simulink model "SRSCrt_MdSwXX_Stat_67_2"  (R2018b)
settings: Solver=FixedStepDiscrete  StartTime=0.0  StopTime=10.0  FixedStep=0.01  RelTol=1e-3
undefined symbols (not defined in the file or in its folder): KeSMSbSRSPosNumConfig_Val
settings Model: Creator=sn2xws  LastModifiedBy=sn2xws
settings DataIOCC: SaveFormat=StructureWithTime
settings OptimizationCC: DefaultParameterBehavior=Inlined  EnhancedBackFolding=on  PassReuseOutputArgsAs=Individual arguments  ZeroExternalMemoryAtStartup=off  ZeroInternalMemoryAtStartup=off  OptimizeBlockOrder=speed  DifferentSizesBufferReuse=on  OptimizationCustomize=off
settings DebuggingCC: ParameterTunabilityLossMsg=error
settings ModelReferenceCC: ModelReferenceNumInstancesAllowed=Single
settings SFSimCC: MATLABDynamicMemAlloc=off
settings RTWCC: SystemTargetFile=autosar.tlc  GenCodeOnly=on  TemplateMakefile=ert_default_tmf  Description=AUTOSAR  GenerateReport=on  IncludeHyperlinkInReport=on  LaunchReport=on  GenerateTraceInfo=on  GenerateTraceReport=on  GenerateTraceReportSl=on  GenerateTraceReportSf=on  GenerateTraceReportEml=on
settings CodeAppCC: ForceParamTrailComments=on  IgnoreCustomStorageClasses=off  OperatorAnnotations=on  SimulinkDataObjDesc=on  SFDataObjDesc=on  InsertBlockDesc=on
settings STFCustomTargetCC: TargetLangStandard=C99 (ISO)  MultiwordLength=256  ParMdlRefBuildCompliant=on  CompOptLevelCompliant=on  IncludeMdlTerminateFcn=off  CombineOutputUpdateFcns=on  SuppressErrorStatus=on  ERTCustomFileBanners=on  SupportNonFinite=off  SupportComplex=off  SupportContinuousTime=off  SupportNonInlinedSFcns=off  RemoveResetFunc=on  MATLABClassNameForMDSCustomization=Simulink.SoftwareTarget.ERTCustomization  AutosarCompliant=on  UseToolchainInfoCompliant=on  LookupTableObjectStructAxisOrder=2,1,3,4,...  LUTObjectStructOrderEvenSpacing=Size,Table,Breakpoints  SystemTargetFile=autosar.tlc
settings ERTTargetCC: TargetLangStandard=C99 (ISO)  ConcurrentExecutionCompliant=off  IncludeMdlTerminateFcn=off  SuppressErrorStatus=on  SupportNonFinite=off  SupportComplex=off  ModelStepFunctionPrototypeControlCompliant=off  CPPClassGenCompliant=off  AutosarCompliant=on  LookupTableObjectStructAxisOrder=2,1,3,4,...  LUTObjectStructOrderEvenSpacing=Size,Table,Breakpoints  InlinedParameterPlacement=NonHierarchical  ERTCustomFileTemplate=example_file_process.tlc

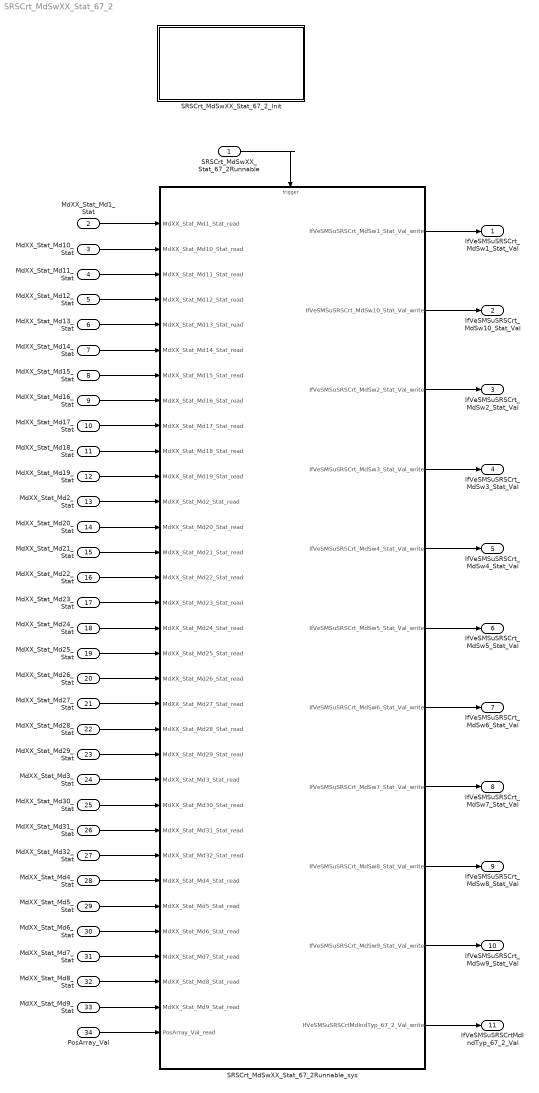
== system SRSCrt_MdSwXX_Stat_67_2 ==
  SRSCrt_MdSwXX_Stat_67_2Runnable : Inport  SampleTime=0.01  OutputFunctionCall=on
  MdXX_Stat_Md1_Stat : Inport  Port=2  OutDataTypeStr=uint8  PortDimensions=1
  MdXX_Stat_Md10_Stat : Inport  Port=3  OutDataTypeStr=uint8  PortDimensions=1
  MdXX_Stat_Md11_Stat : Inport  Port=4  OutDataTypeStr=uint8  PortDimensions=1
  MdXX_Stat_Md12_Stat : Inport  Port=5  OutDataTypeStr=uint8  PortDimensions=1
  MdXX_Stat_Md13_Stat : Inport  Port=6  OutDataTypeStr=uint8  PortDimensions=1
  MdXX_Stat_Md14_Stat : Inport  Port=7  OutDataTypeStr=uint8  PortDimensions=1
  MdXX_Stat_Md15_Stat : Inport  Port=8  OutDataTypeStr=uint8  PortDimensions=1
  MdXX_Stat_Md16_Stat : Inport  Port=9  OutDataTypeStr=uint8  PortDimensions=1
  MdXX_Stat_Md17_Stat : Inport  Port=10  OutDataTypeStr=uint8  PortDimensions=1
  MdXX_Stat_Md18_Stat : Inport  Port=11  OutDataTypeStr=uint8  PortDimensions=1
  MdXX_Stat_Md19_Stat : Inport  Port=12  OutDataTypeStr=uint8  PortDimensions=1
  MdXX_Stat_Md2_Stat : Inport  Port=13  OutDataTypeStr=uint8  PortDimensions=1
  MdXX_Stat_Md20_Stat : Inport  Port=14  OutDataTypeStr=uint8  PortDimensions=1
  MdXX_Stat_Md21_Stat : Inport  Port=15  OutDataTypeStr=uint8  PortDimensions=1
  MdXX_Stat_Md22_Stat : Inport  Port=16  OutDataTypeStr=uint8  PortDimensions=1
  MdXX_Stat_Md23_Stat : Inport  Port=17  OutDataTypeStr=uint8  PortDimensions=1
  MdXX_Stat_Md24_Stat : Inport  Port=18  OutDataTypeStr=uint8  PortDimensions=1
  MdXX_Stat_Md25_Stat : Inport  Port=19  OutDataTypeStr=uint8  PortDimensions=1
  MdXX_Stat_Md26_Stat : Inport  Port=20  OutDataTypeStr=uint8  PortDimensions=1
  MdXX_Stat_Md27_Stat : Inport  Port=21  OutDataTypeStr=uint8  PortDimensions=1
  MdXX_Stat_Md28_Stat : Inport  Port=22  OutDataTypeStr=uint8  PortDimensions=1
  MdXX_Stat_Md29_Stat : Inport  Port=23  OutDataTypeStr=uint8  PortDimensions=1
  MdXX_Stat_Md3_Stat : Inport  Port=24  OutDataTypeStr=uint8  PortDimensions=1
  MdXX_Stat_Md30_Stat : Inport  Port=25  OutDataTypeStr=uint8  PortDimensions=1
  MdXX_Stat_Md31_Stat : Inport  Port=26  OutDataTypeStr=uint8  PortDimensions=1
  MdXX_Stat_Md32_Stat : Inport  Port=27  OutDataTypeStr=uint8  PortDimensions=1
  MdXX_Stat_Md4_Stat : Inport  Port=28  OutDataTypeStr=uint8  PortDimensions=1
  MdXX_Stat_Md5_Stat : Inport  Port=29  OutDataTypeStr=uint8  PortDimensions=1
  MdXX_Stat_Md6_Stat : Inport  Port=30  OutDataTypeStr=uint8  PortDimensions=1
  MdXX_Stat_Md7_Stat : Inport  Port=31  OutDataTypeStr=uint8  PortDimensions=1
  MdXX_Stat_Md8_Stat : Inport  Port=32  OutDataTypeStr=uint8  PortDimensions=1
  MdXX_Stat_Md9_Stat : Inport  Port=33  OutDataTypeStr=uint8  PortDimensions=1
  PosArray_Val : Inport  Port=34  OutDataTypeStr=uint8  PortDimensions=11
  SRSCrt_MdSwXX_Stat_67_2Runnable_sys : Subsystem
  SRSCrt_MdSwXX_Stat_67_2_Init : Subsystem
  IfVeSMSuSRSCrt_MdSw1_Stat_Val : Outport  OutDataTypeStr=uint8  PortDimensions=1
  IfVeSMSuSRSCrt_MdSw10_Stat_Val : Outport  Port=2  OutDataTypeStr=uint8  PortDimensions=1
  IfVeSMSuSRSCrt_MdSw2_Stat_Val : Outport  Port=3  OutDataTypeStr=uint8  PortDimensions=1
  IfVeSMSuSRSCrt_MdSw3_Stat_Val : Outport  Port=4  OutDataTypeStr=uint8  PortDimensions=1
  IfVeSMSuSRSCrt_MdSw4_Stat_Val : Outport  Port=5  OutDataTypeStr=uint8  PortDimensions=1
  IfVeSMSuSRSCrt_MdSw5_Stat_Val : Outport  Port=6  OutDataTypeStr=uint8  PortDimensions=1
  IfVeSMSuSRSCrt_MdSw6_Stat_Val : Outport  Port=7  OutDataTypeStr=uint8  PortDimensions=1
  IfVeSMSuSRSCrt_MdSw7_Stat_Val : Outport  Port=8  OutDataTypeStr=uint8  PortDimensions=1
  IfVeSMSuSRSCrt_MdSw8_Stat_Val : Outport  Port=9  OutDataTypeStr=uint8  PortDimensions=1
  IfVeSMSuSRSCrt_MdSw9_Stat_Val : Outport  Port=10  OutDataTypeStr=uint8  PortDimensions=1
  IfVeSMSuSRSCrtMdIndTyp_67_2_Val : Outport  Port=11  OutDataTypeStr=uint8  PortDimensions=1
  wires:
  MdXX_Stat_Md1_Stat/1 -> SRSCrt_MdSwXX_Stat_67_2Runnable_sys/1(MdXX_Stat_Md1_Stat_read)
  MdXX_Stat_Md10_Stat/1 -> SRSCrt_MdSwXX_Stat_67_2Runnable_sys/2(MdXX_Stat_Md10_Stat_read)
  MdXX_Stat_Md11_Stat/1 -> SRSCrt_MdSwXX_Stat_67_2Runnable_sys/3(MdXX_Stat_Md11_Stat_read)
  MdXX_Stat_Md12_Stat/1 -> SRSCrt_MdSwXX_Stat_67_2Runnable_sys/4(MdXX_Stat_Md12_Stat_read)
  MdXX_Stat_Md13_Stat/1 -> SRSCrt_MdSwXX_Stat_67_2Runnable_sys/5(MdXX_Stat_Md13_Stat_read)
  MdXX_Stat_Md14_Stat/1 -> SRSCrt_MdSwXX_Stat_67_2Runnable_sys/6(MdXX_Stat_Md14_Stat_read)
  MdXX_Stat_Md15_Stat/1 -> SRSCrt_MdSwXX_Stat_67_2Runnable_sys/7(MdXX_Stat_Md15_Stat_read)
  MdXX_Stat_Md16_Stat/1 -> SRSCrt_MdSwXX_Stat_67_2Runnable_sys/8(MdXX_Stat_Md16_Stat_read)
  MdXX_Stat_Md17_Stat/1 -> SRSCrt_MdSwXX_Stat_67_2Runnable_sys/9(MdXX_Stat_Md17_Stat_read)
  MdXX_Stat_Md18_Stat/1 -> SRSCrt_MdSwXX_Stat_67_2Runnable_sys/10(MdXX_Stat_Md18_Stat_read)
  MdXX_Stat_Md19_Stat/1 -> SRSCrt_MdSwXX_Stat_67_2Runnable_sys/11(MdXX_Stat_Md19_Stat_read)
  MdXX_Stat_Md2_Stat/1 -> SRSCrt_MdSwXX_Stat_67_2Runnable_sys/12(MdXX_Stat_Md2_Stat_read)
  MdXX_Stat_Md20_Stat/1 -> SRSCrt_MdSwXX_Stat_67_2Runnable_sys/13(MdXX_Stat_Md20_Stat_read)
  MdXX_Stat_Md21_Stat/1 -> SRSCrt_MdSwXX_Stat_67_2Runnable_sys/14(MdXX_Stat_Md21_Stat_read)
  MdXX_Stat_Md22_Stat/1 -> SRSCrt_MdSwXX_Stat_67_2Runnable_sys/15(MdXX_Stat_Md22_Stat_read)
  MdXX_Stat_Md23_Stat/1 -> SRSCrt_MdSwXX_Stat_67_2Runnable_sys/16(MdXX_Stat_Md23_Stat_read)
  MdXX_Stat_Md24_Stat/1 -> SRSCrt_MdSwXX_Stat_67_2Runnable_sys/17(MdXX_Stat_Md24_Stat_read)
  MdXX_Stat_Md25_Stat/1 -> SRSCrt_MdSwXX_Stat_67_2Runnable_sys/18(MdXX_Stat_Md25_Stat_read)
  MdXX_Stat_Md26_Stat/1 -> SRSCrt_MdSwXX_Stat_67_2Runnable_sys/19(MdXX_Stat_Md26_Stat_read)
  MdXX_Stat_Md27_Stat/1 -> SRSCrt_MdSwXX_Stat_67_2Runnable_sys/20(MdXX_Stat_Md27_Stat_read)
  MdXX_Stat_Md28_Stat/1 -> SRSCrt_MdSwXX_Stat_67_2Runnable_sys/21(MdXX_Stat_Md28_Stat_read)
  MdXX_Stat_Md29_Stat/1 -> SRSCrt_MdSwXX_Stat_67_2Runnable_sys/22(MdXX_Stat_Md29_Stat_read)
  MdXX_Stat_Md3_Stat/1 -> SRSCrt_MdSwXX_Stat_67_2Runnable_sys/23(MdXX_Stat_Md3_Stat_read)
  MdXX_Stat_Md30_Stat/1 -> SRSCrt_MdSwXX_Stat_67_2Runnable_sys/24(MdXX_Stat_Md30_Stat_read)
  MdXX_Stat_Md31_Stat/1 -> SRSCrt_MdSwXX_Stat_67_2Runnable_sys/25(MdXX_Stat_Md31_Stat_read)
  MdXX_Stat_Md32_Stat/1 -> SRSCrt_MdSwXX_Stat_67_2Runnable_sys/26(MdXX_Stat_Md32_Stat_read)
  MdXX_Stat_Md4_Stat/1 -> SRSCrt_MdSwXX_Stat_67_2Runnable_sys/27(MdXX_Stat_Md4_Stat_read)
  MdXX_Stat_Md5_Stat/1 -> SRSCrt_MdSwXX_Stat_67_2Runnable_sys/28(MdXX_Stat_Md5_Stat_read)
  MdXX_Stat_Md6_Stat/1 -> SRSCrt_MdSwXX_Stat_67_2Runnable_sys/29(MdXX_Stat_Md6_Stat_read)
  MdXX_Stat_Md7_Stat/1 -> SRSCrt_MdSwXX_Stat_67_2Runnable_sys/30(MdXX_Stat_Md7_Stat_read)
  MdXX_Stat_Md8_Stat/1 -> SRSCrt_MdSwXX_Stat_67_2Runnable_sys/31(MdXX_Stat_Md8_Stat_read)
  MdXX_Stat_Md9_Stat/1 -> SRSCrt_MdSwXX_Stat_67_2Runnable_sys/32(MdXX_Stat_Md9_Stat_read)
  PosArray_Val/1 -> SRSCrt_MdSwXX_Stat_67_2Runnable_sys/33(PosArray_Val_read)
  SRSCrt_MdSwXX_Stat_67_2Runnable_sys/1(IfVeSMSuSRSCrt_MdSw1_Stat_Val_write) -> IfVeSMSuSRSCrt_MdSw1_Stat_Val/1
  SRSCrt_MdSwXX_Stat_67_2Runnable_sys/2(IfVeSMSuSRSCrt_MdSw10_Stat_Val_write) -> IfVeSMSuSRSCrt_MdSw10_Stat_Val/1
  SRSCrt_MdSwXX_Stat_67_2Runnable_sys/3(IfVeSMSuSRSCrt_MdSw2_Stat_Val_write) -> IfVeSMSuSRSCrt_MdSw2_Stat_Val/1
  SRSCrt_MdSwXX_Stat_67_2Runnable_sys/4(IfVeSMSuSRSCrt_MdSw3_Stat_Val_write) -> IfVeSMSuSRSCrt_MdSw3_Stat_Val/1
  SRSCrt_MdSwXX_Stat_67_2Runnable_sys/5(IfVeSMSuSRSCrt_MdSw4_Stat_Val_write) -> IfVeSMSuSRSCrt_MdSw4_Stat_Val/1
  SRSCrt_MdSwXX_Stat_67_2Runnable_sys/6(IfVeSMSuSRSCrt_MdSw5_Stat_Val_write) -> IfVeSMSuSRSCrt_MdSw5_Stat_Val/1
  SRSCrt_MdSwXX_Stat_67_2Runnable_sys/7(IfVeSMSuSRSCrt_MdSw6_Stat_Val_write) -> IfVeSMSuSRSCrt_MdSw6_Stat_Val/1
  SRSCrt_MdSwXX_Stat_67_2Runnable_sys/8(IfVeSMSuSRSCrt_MdSw7_Stat_Val_write) -> IfVeSMSuSRSCrt_MdSw7_Stat_Val/1
  SRSCrt_MdSwXX_Stat_67_2Runnable_sys/9(IfVeSMSuSRSCrt_MdSw8_Stat_Val_write) -> IfVeSMSuSRSCrt_MdSw8_Stat_Val/1
  SRSCrt_MdSwXX_Stat_67_2Runnable_sys/10(IfVeSMSuSRSCrt_MdSw9_Stat_Val_write) -> IfVeSMSuSRSCrt_MdSw9_Stat_Val/1
  SRSCrt_MdSwXX_Stat_67_2Runnable_sys/11(IfVeSMSuSRSCrtMdIndTyp_67_2_Val_write) -> IfVeSMSuSRSCrtMdIndTyp_67_2_Val/1
  SRSCrt_MdSwXX_Stat_67_2Runnable/1 -> SRSCrt_MdSwXX_Stat_67_2Runnable_sys/Trigger

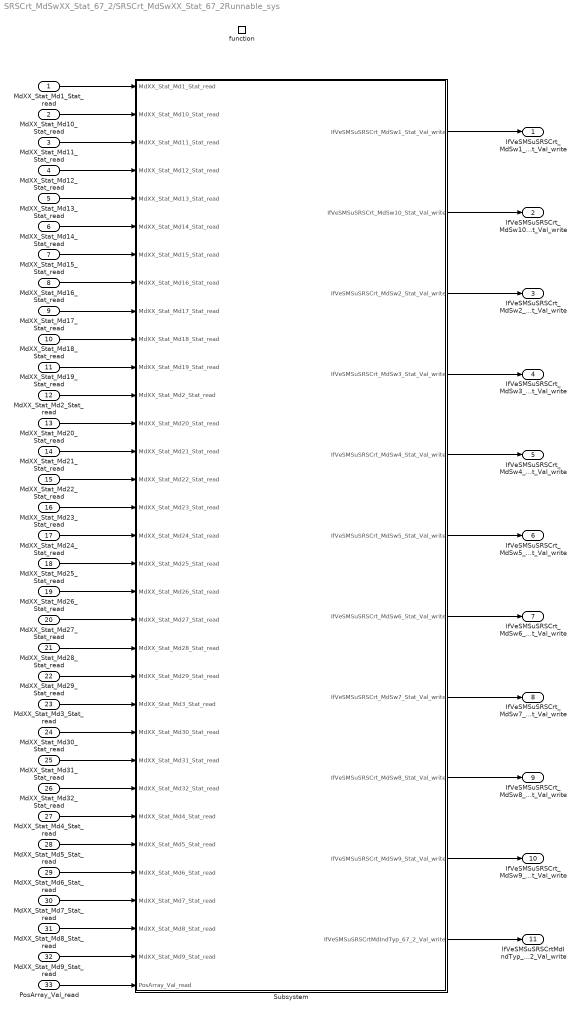
== system SRSCrt_MdSwXX_Stat_67_2/SRSCrt_MdSwXX_Stat_67_2Runnable_sys ==
  MdXX_Stat_Md1_Stat_read : Inport
  MdXX_Stat_Md10_Stat_read : Inport  Port=2
  MdXX_Stat_Md11_Stat_read : Inport  Port=3
  MdXX_Stat_Md12_Stat_read : Inport  Port=4
  MdXX_Stat_Md13_Stat_read : Inport  Port=5
  MdXX_Stat_Md14_Stat_read : Inport  Port=6
  MdXX_Stat_Md15_Stat_read : Inport  Port=7
  MdXX_Stat_Md16_Stat_read : Inport  Port=8
  MdXX_Stat_Md17_Stat_read : Inport  Port=9
  MdXX_Stat_Md18_Stat_read : Inport  Port=10
  MdXX_Stat_Md19_Stat_read : Inport  Port=11
  MdXX_Stat_Md2_Stat_read : Inport  Port=12
  MdXX_Stat_Md20_Stat_read : Inport  Port=13
  MdXX_Stat_Md21_Stat_read : Inport  Port=14
  MdXX_Stat_Md22_Stat_read : Inport  Port=15
  MdXX_Stat_Md23_Stat_read : Inport  Port=16
  MdXX_Stat_Md24_Stat_read : Inport  Port=17
  MdXX_Stat_Md25_Stat_read : Inport  Port=18
  MdXX_Stat_Md26_Stat_read : Inport  Port=19
  MdXX_Stat_Md27_Stat_read : Inport  Port=20
  MdXX_Stat_Md28_Stat_read : Inport  Port=21
  MdXX_Stat_Md29_Stat_read : Inport  Port=22
  MdXX_Stat_Md3_Stat_read : Inport  Port=23
  MdXX_Stat_Md30_Stat_read : Inport  Port=24
  MdXX_Stat_Md31_Stat_read : Inport  Port=25
  MdXX_Stat_Md32_Stat_read : Inport  Port=26
  MdXX_Stat_Md4_Stat_read : Inport  Port=27
  MdXX_Stat_Md5_Stat_read : Inport  Port=28
  MdXX_Stat_Md6_Stat_read : Inport  Port=29
  MdXX_Stat_Md7_Stat_read : Inport  Port=30
  MdXX_Stat_Md8_Stat_read : Inport  Port=31
  MdXX_Stat_Md9_Stat_read : Inport  Port=32
  PosArray_Val_read : Inport  Port=33
  function : TriggerPort  TriggerType=function-call  VariantControl=(inherit)  SampleTimeType=periodic  SampleTime=-1
  Subsystem : Subsystem
  IfVeSMSuSRSCrt_MdSw1_Stat_Val_write : Outport
  IfVeSMSuSRSCrt_MdSw10_Stat_Val_write : Outport  Port=2
  IfVeSMSuSRSCrt_MdSw2_Stat_Val_write : Outport  Port=3
  IfVeSMSuSRSCrt_MdSw3_Stat_Val_write : Outport  Port=4
  IfVeSMSuSRSCrt_MdSw4_Stat_Val_write : Outport  Port=5
  IfVeSMSuSRSCrt_MdSw5_Stat_Val_write : Outport  Port=6
  IfVeSMSuSRSCrt_MdSw6_Stat_Val_write : Outport  Port=7
  IfVeSMSuSRSCrt_MdSw7_Stat_Val_write : Outport  Port=8
  IfVeSMSuSRSCrt_MdSw8_Stat_Val_write : Outport  Port=9
  IfVeSMSuSRSCrt_MdSw9_Stat_Val_write : Outport  Port=10
  IfVeSMSuSRSCrtMdIndTyp_67_2_Val_write : Outport  Port=11
  wires:
  MdXX_Stat_Md1_Stat_read/1 -> Subsystem/1(MdXX_Stat_Md1_Stat_read)
  MdXX_Stat_Md10_Stat_read/1 -> Subsystem/2(MdXX_Stat_Md10_Stat_read)
  MdXX_Stat_Md11_Stat_read/1 -> Subsystem/3(MdXX_Stat_Md11_Stat_read)
  MdXX_Stat_Md12_Stat_read/1 -> Subsystem/4(MdXX_Stat_Md12_Stat_read)
  MdXX_Stat_Md13_Stat_read/1 -> Subsystem/5(MdXX_Stat_Md13_Stat_read)
  MdXX_Stat_Md14_Stat_read/1 -> Subsystem/6(MdXX_Stat_Md14_Stat_read)
  MdXX_Stat_Md15_Stat_read/1 -> Subsystem/7(MdXX_Stat_Md15_Stat_read)
  MdXX_Stat_Md16_Stat_read/1 -> Subsystem/8(MdXX_Stat_Md16_Stat_read)
  MdXX_Stat_Md17_Stat_read/1 -> Subsystem/9(MdXX_Stat_Md17_Stat_read)
  MdXX_Stat_Md18_Stat_read/1 -> Subsystem/10(MdXX_Stat_Md18_Stat_read)
  MdXX_Stat_Md19_Stat_read/1 -> Subsystem/11(MdXX_Stat_Md19_Stat_read)
  MdXX_Stat_Md2_Stat_read/1 -> Subsystem/12(MdXX_Stat_Md2_Stat_read)
  MdXX_Stat_Md20_Stat_read/1 -> Subsystem/13(MdXX_Stat_Md20_Stat_read)
  MdXX_Stat_Md21_Stat_read/1 -> Subsystem/14(MdXX_Stat_Md21_Stat_read)
  MdXX_Stat_Md22_Stat_read/1 -> Subsystem/15(MdXX_Stat_Md22_Stat_read)
  MdXX_Stat_Md23_Stat_read/1 -> Subsystem/16(MdXX_Stat_Md23_Stat_read)
  MdXX_Stat_Md24_Stat_read/1 -> Subsystem/17(MdXX_Stat_Md24_Stat_read)
  MdXX_Stat_Md25_Stat_read/1 -> Subsystem/18(MdXX_Stat_Md25_Stat_read)
  MdXX_Stat_Md26_Stat_read/1 -> Subsystem/19(MdXX_Stat_Md26_Stat_read)
  MdXX_Stat_Md27_Stat_read/1 -> Subsystem/20(MdXX_Stat_Md27_Stat_read)
  MdXX_Stat_Md28_Stat_read/1 -> Subsystem/21(MdXX_Stat_Md28_Stat_read)
  MdXX_Stat_Md29_Stat_read/1 -> Subsystem/22(MdXX_Stat_Md29_Stat_read)
  MdXX_Stat_Md3_Stat_read/1 -> Subsystem/23(MdXX_Stat_Md3_Stat_read)
  MdXX_Stat_Md30_Stat_read/1 -> Subsystem/24(MdXX_Stat_Md30_Stat_read)
  MdXX_Stat_Md31_Stat_read/1 -> Subsystem/25(MdXX_Stat_Md31_Stat_read)
  MdXX_Stat_Md32_Stat_read/1 -> Subsystem/26(MdXX_Stat_Md32_Stat_read)
  MdXX_Stat_Md4_Stat_read/1 -> Subsystem/27(MdXX_Stat_Md4_Stat_read)
  MdXX_Stat_Md5_Stat_read/1 -> Subsystem/28(MdXX_Stat_Md5_Stat_read)
  MdXX_Stat_Md6_Stat_read/1 -> Subsystem/29(MdXX_Stat_Md6_Stat_read)
  MdXX_Stat_Md7_Stat_read/1 -> Subsystem/30(MdXX_Stat_Md7_Stat_read)
  MdXX_Stat_Md8_Stat_read/1 -> Subsystem/31(MdXX_Stat_Md8_Stat_read)
  MdXX_Stat_Md9_Stat_read/1 -> Subsystem/32(MdXX_Stat_Md9_Stat_read)
  PosArray_Val_read/1 -> Subsystem/33(PosArray_Val_read)
  Subsystem/1(IfVeSMSuSRSCrt_MdSw1_Stat_Val_write) -> IfVeSMSuSRSCrt_MdSw1_Stat_Val_write/1
  Subsystem/2(IfVeSMSuSRSCrt_MdSw10_Stat_Val_write) -> IfVeSMSuSRSCrt_MdSw10_Stat_Val_write/1
  Subsystem/3(IfVeSMSuSRSCrt_MdSw2_Stat_Val_write) -> IfVeSMSuSRSCrt_MdSw2_Stat_Val_write/1
  Subsystem/4(IfVeSMSuSRSCrt_MdSw3_Stat_Val_write) -> IfVeSMSuSRSCrt_MdSw3_Stat_Val_write/1
  Subsystem/5(IfVeSMSuSRSCrt_MdSw4_Stat_Val_write) -> IfVeSMSuSRSCrt_MdSw4_Stat_Val_write/1
  Subsystem/6(IfVeSMSuSRSCrt_MdSw5_Stat_Val_write) -> IfVeSMSuSRSCrt_MdSw5_Stat_Val_write/1
  Subsystem/7(IfVeSMSuSRSCrt_MdSw6_Stat_Val_write) -> IfVeSMSuSRSCrt_MdSw6_Stat_Val_write/1
  Subsystem/8(IfVeSMSuSRSCrt_MdSw7_Stat_Val_write) -> IfVeSMSuSRSCrt_MdSw7_Stat_Val_write/1
  Subsystem/9(IfVeSMSuSRSCrt_MdSw8_Stat_Val_write) -> IfVeSMSuSRSCrt_MdSw8_Stat_Val_write/1
  Subsystem/10(IfVeSMSuSRSCrt_MdSw9_Stat_Val_write) -> IfVeSMSuSRSCrt_MdSw9_Stat_Val_write/1
  Subsystem/11(IfVeSMSuSRSCrtMdIndTyp_67_2_Val_write) -> IfVeSMSuSRSCrtMdIndTyp_67_2_Val_write/1

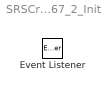
== system SRSCrt_MdSwXX_Stat_67_2/SRSCrt_MdSwXX_Stat_67_2_Init ==
  Event Listener : EventListener  EventName=reset

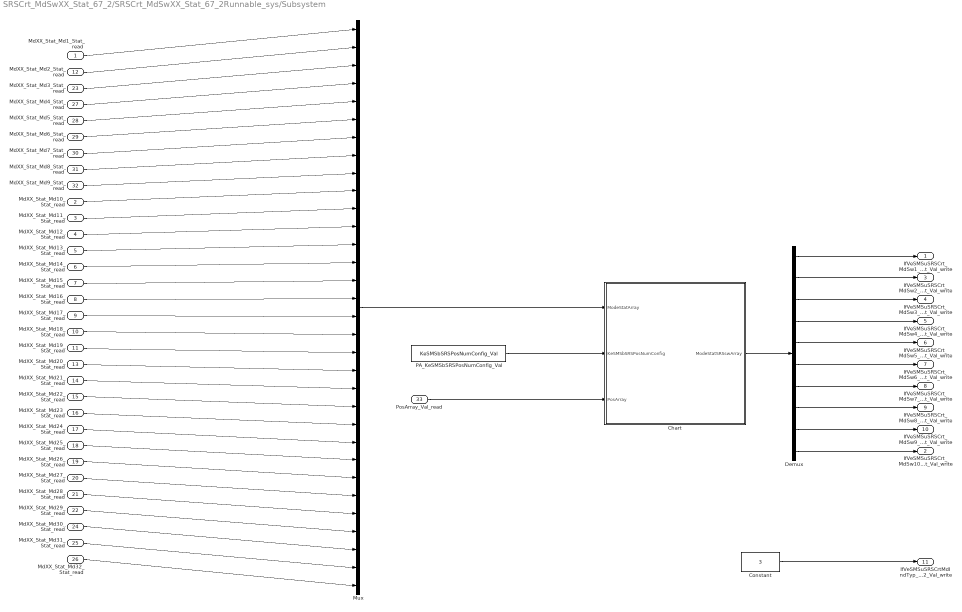
== system SRSCrt_MdSwXX_Stat_67_2/SRSCrt_MdSwXX_Stat_67_2Runnable_sys/Subsystem ==
  MdXX_Stat_Md1_Stat_read : Inport
  MdXX_Stat_Md10_Stat_read : Inport  Port=2
  MdXX_Stat_Md11_Stat_read : Inport  Port=3
  MdXX_Stat_Md12_Stat_read : Inport  Port=4
  MdXX_Stat_Md13_Stat_read : Inport  Port=5
  MdXX_Stat_Md14_Stat_read : Inport  Port=6
  MdXX_Stat_Md15_Stat_read : Inport  Port=7
  MdXX_Stat_Md16_Stat_read : Inport  Port=8
  MdXX_Stat_Md17_Stat_read : Inport  Port=9
  MdXX_Stat_Md18_Stat_read : Inport  Port=10
  MdXX_Stat_Md19_Stat_read : Inport  Port=11
  MdXX_Stat_Md2_Stat_read : Inport  Port=12
  MdXX_Stat_Md20_Stat_read : Inport  Port=13
  MdXX_Stat_Md21_Stat_read : Inport  Port=14
  MdXX_Stat_Md22_Stat_read : Inport  Port=15
  MdXX_Stat_Md23_Stat_read : Inport  Port=16
  MdXX_Stat_Md24_Stat_read : Inport  Port=17
  MdXX_Stat_Md25_Stat_read : Inport  Port=18
  MdXX_Stat_Md26_Stat_read : Inport  Port=19
  MdXX_Stat_Md27_Stat_read : Inport  Port=20
  MdXX_Stat_Md28_Stat_read : Inport  Port=21
  MdXX_Stat_Md29_Stat_read : Inport  Port=22
  MdXX_Stat_Md3_Stat_read : Inport  Port=23
  MdXX_Stat_Md30_Stat_read : Inport  Port=24
  MdXX_Stat_Md31_Stat_read : Inport  Port=25
  MdXX_Stat_Md32_Stat_read : Inport  Port=26
  MdXX_Stat_Md4_Stat_read : Inport  Port=27
  MdXX_Stat_Md5_Stat_read : Inport  Port=28
  MdXX_Stat_Md6_Stat_read : Inport  Port=29
  MdXX_Stat_Md7_Stat_read : Inport  Port=30
  MdXX_Stat_Md8_Stat_read : Inport  Port=31
  MdXX_Stat_Md9_Stat_read : Inport  Port=32
  PosArray_Val_read : Inport  Port=33
  Chart : Stateflow chart  TreatAsAtomicUnit=on
  Constant : Constant  Value=3  OutDataTypeStr=uint8
  Demux : Demux  Outputs=10
  Mux : Mux  Inputs=32
  PA_KeSMSbSRSPosNumConfig_Val : Constant  Value=KeSMSbSRSPosNumConfig_Val
  IfVeSMSuSRSCrt_MdSw1_Stat_Val_write : Outport
      settings: EnsureOutportIsVirtual=on
  IfVeSMSuSRSCrt_MdSw10_Stat_Val_write : Outport  Port=2
      settings: EnsureOutportIsVirtual=on
  IfVeSMSuSRSCrt_MdSw2_Stat_Val_write : Outport  Port=3
      settings: EnsureOutportIsVirtual=on
  IfVeSMSuSRSCrt_MdSw3_Stat_Val_write : Outport  Port=4
      settings: EnsureOutportIsVirtual=on
  IfVeSMSuSRSCrt_MdSw4_Stat_Val_write : Outport  Port=5
      settings: EnsureOutportIsVirtual=on
  IfVeSMSuSRSCrt_MdSw5_Stat_Val_write : Outport  Port=6
      settings: EnsureOutportIsVirtual=on
  IfVeSMSuSRSCrt_MdSw6_Stat_Val_write : Outport  Port=7
      settings: EnsureOutportIsVirtual=on
  IfVeSMSuSRSCrt_MdSw7_Stat_Val_write : Outport  Port=8
      settings: EnsureOutportIsVirtual=on
  IfVeSMSuSRSCrt_MdSw8_Stat_Val_write : Outport  Port=9
      settings: EnsureOutportIsVirtual=on
  IfVeSMSuSRSCrt_MdSw9_Stat_Val_write : Outport  Port=10
      settings: EnsureOutportIsVirtual=on
  IfVeSMSuSRSCrtMdIndTyp_67_2_Val_write : Outport  Port=11
      settings: EnsureOutportIsVirtual=on
  wires:
  Mux/1 -> Chart/1(ModeStatArray)
  PosArray_Val_read/1 -> Chart/3(PosArray)
  PA_KeSMSbSRSPosNumConfig_Val/1 -> Chart/2(KeSMSbSRSPosNumConfig)
  Chart/1(ModeStatSRSswArray) -> Demux/1
  Demux/2 -> IfVeSMSuSRSCrt_MdSw2_Stat_Val_write/1
  Demux/3 -> IfVeSMSuSRSCrt_MdSw3_Stat_Val_write/1
  Demux/4 -> IfVeSMSuSRSCrt_MdSw4_Stat_Val_write/1
  Demux/5 -> IfVeSMSuSRSCrt_MdSw5_Stat_Val_write/1
  Demux/6 -> IfVeSMSuSRSCrt_MdSw6_Stat_Val_write/1
  Demux/7 -> IfVeSMSuSRSCrt_MdSw7_Stat_Val_write/1
  Demux/8 -> IfVeSMSuSRSCrt_MdSw8_Stat_Val_write/1
  Demux/9 -> IfVeSMSuSRSCrt_MdSw9_Stat_Val_write/1
  Demux/10 -> IfVeSMSuSRSCrt_MdSw10_Stat_Val_write/1
  Demux/1 -> IfVeSMSuSRSCrt_MdSw1_Stat_Val_write/1
  MdXX_Stat_Md1_Stat_read/1 -> Mux/1
  MdXX_Stat_Md2_Stat_read/1 -> Mux/2
  MdXX_Stat_Md3_Stat_read/1 -> Mux/3
  MdXX_Stat_Md4_Stat_read/1 -> Mux/4
  MdXX_Stat_Md5_Stat_read/1 -> Mux/5
  MdXX_Stat_Md6_Stat_read/1 -> Mux/6
  MdXX_Stat_Md7_Stat_read/1 -> Mux/7
  MdXX_Stat_Md8_Stat_read/1 -> Mux/8
  MdXX_Stat_Md9_Stat_read/1 -> Mux/9
  MdXX_Stat_Md10_Stat_read/1 -> Mux/10
  MdXX_Stat_Md11_Stat_read/1 -> Mux/11
  MdXX_Stat_Md12_Stat_read/1 -> Mux/12
  MdXX_Stat_Md13_Stat_read/1 -> Mux/13
  MdXX_Stat_Md14_Stat_read/1 -> Mux/14
  MdXX_Stat_Md15_Stat_read/1 -> Mux/15
  MdXX_Stat_Md16_Stat_read/1 -> Mux/16
  MdXX_Stat_Md17_Stat_read/1 -> Mux/17
  MdXX_Stat_Md18_Stat_read/1 -> Mux/18
  MdXX_Stat_Md19_Stat_read/1 -> Mux/19
  MdXX_Stat_Md20_Stat_read/1 -> Mux/20
  MdXX_Stat_Md21_Stat_read/1 -> Mux/21
  MdXX_Stat_Md22_Stat_read/1 -> Mux/22
  MdXX_Stat_Md23_Stat_read/1 -> Mux/23
  MdXX_Stat_Md24_Stat_read/1 -> Mux/24
  MdXX_Stat_Md25_Stat_read/1 -> Mux/25
  MdXX_Stat_Md26_Stat_read/1 -> Mux/26
  MdXX_Stat_Md27_Stat_read/1 -> Mux/27
  MdXX_Stat_Md28_Stat_read/1 -> Mux/28
  MdXX_Stat_Md29_Stat_read/1 -> Mux/29
  MdXX_Stat_Md30_Stat_read/1 -> Mux/30
  MdXX_Stat_Md31_Stat_read/1 -> Mux/31
  MdXX_Stat_Md32_Stat_read/1 -> Mux/32
  Constant/1 -> IfVeSMSuSRSCrtMdIndTyp_67_2_Val_write/1

== stateflow chart SRSCrt_MdSwXX_Stat_67_2/SRSCrt_MdSwXX_Stat_67_2Runnable_sys/Subsystem/Chart ==
  (default) -> (junction 5) : {i=0;}
  (junction 7) -> (junction 22) [order 1] : [PosArray[i+1]<1]
  (junction 5) -> (junction 7) [order 1] : [i<KeSMSbSRSPosNumConfig]
  (junction 7) -> (junction 9) [order 2] : {
      | ModeStatSRSswArray[i]=ModeStatArray[PosArray[i+1]-1];
      | }
  (junction 22) -> (junction 24) : {
      | ModeStatSRSswArray[i]=0;
      | }
  (junction 9) -> (junction 5) : {i=i+1;}
  (junction 5) -> (junction 12) [order 2]
  (junction 24) -> (junction 9)
  (junction 12) -> (junction 14) [order 1] : [i<10]
  (junction 14) -> (junction 16) : {
      | ModeStatSRSswArray[i]=0;
      | }
  (junction 16) -> (junction 12) : {i=i+1;}
  (junction 12) -> (junction 19) [order 2]
  data: ModeStatArray input uint8 size=32; KeSMSbSRSPosNumConfig input uint8; i local uint8; ModeStatSRSswArray output uint8 size=10; PosArray input uint8 size=11
